simulink model "SignalDistributor"  (R2022a)
settings: Solver=VariableStepAuto  StartTime=0.0  StopTime=10.0  RelTol=1e-3
settings Model: Creator=Lenovo  LastModifiedBy=Lenovo

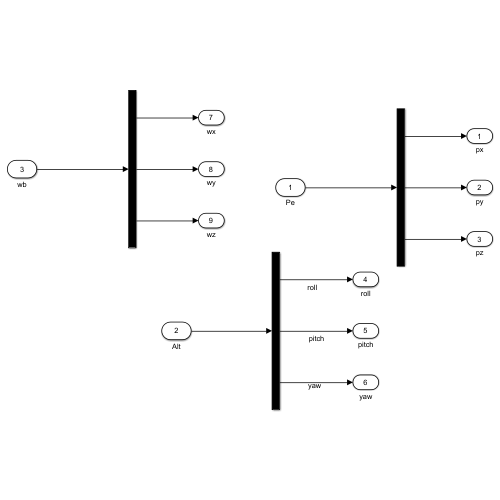
[thumbnail: Simulink's stored preview of the top-level diagram]
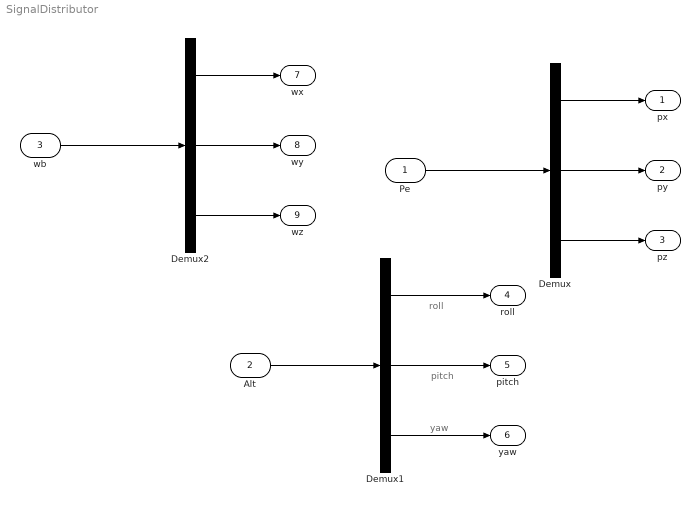
== system SignalDistributor ==
  note: yaw
  note: pitch
  note: roll
  Pe : Inport
  Alt : Inport  Port=2
  wb : Inport  Port=3
  Demux : Demux  Outputs=3
  Demux1 : Demux  Outputs=3
  Demux2 : Demux  Outputs=3
  px : Outport
  py : Outport  Port=2
  pz : Outport  Port=3
  roll : Outport  Port=4
  pitch : Outport  Port=5
  yaw : Outport  Port=6
  wx : Outport  Port=7
  wy : Outport  Port=8
  wz : Outport  Port=9
  wires:
  Demux/1 -> px/1
  Demux/2 -> py/1
  Demux/3 -> pz/1
  Pe/1 -> Demux/1
  Alt/1 -> Demux1/1
  Demux1/3 -> yaw/1
  Demux1/2 -> pitch/1
  Demux1/1 -> roll/1
  Demux2/1 -> wx/1
  Demux2/2 -> wy/1
  Demux2/3 -> wz/1
  wb/1 -> Demux2/1
